simulink library "engine_AMT280_lib"  (Simulink 7.2)
settings: Solver=ode45  SolverMode=SingleTasking  StartTime=0.0  StopTime=10.0  RelTol=1e-3
libraries: simulink x1
settings Model: Creator=amurch  LastModifiedBy=amurch

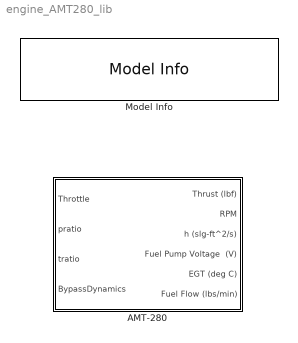
== system engine_AMT280_lib ==
  AMT-280 : Subsystem
      mask init:
      | % Curve fit parameters for AMT-280 Model
      | Coeff_thrust   = [ 5.7372e-05  -5.2629e-03   3.1586e-01  -5.1517e+00];
      | Coeff_throttle = [ -4.3078e-03   1.1110e+00   2.9012e+01];
      | Coeff_fuelflow = [ 1.0140e-04  -1.5867e-03   2.0125e-01];
      | Coeff_tau      = [ -2.2400e-02   2.9948e+00];
      | 
      | 
      | % Equvalent Shaft parameters for engine
      | shaft_dia = 0.75/12.0;       % diameter of rotating turbine in feet 
      | shaft_len = 6.25/12.0;       % length of rotating turbine in feet   
      | density   = 15.2;            % mass density of steel in slugs/ft^3 
      | 
      | fuelpump_table = [ 0.90 1.0 6.4]; %volts, table of fuel pump voltages  - not accurate at the moment 2-4-08
      | fuelflow_table = [0.00 0.1762 1.34044]; %lbs/min,   fuel flow rates corresponding to pump voltages (pumpv_table)
  Model Info : simulink/Model-Wide Utilities/Model Info  SystemSampleTime=-1  InitialBlockCM=None  BlockCM=None  Frame=on  DisplayStringWithTags=|  HorizontalTextAlignment=Center  LeftAlignmentValue=0.5  SourceBlockDiagram=engine_AMT280_lib  TagMaxNumber=20
      | AMT-280 Engine Library
      | 
      | Model Version: %<ModelVersion>
      | Last modifed by %<LastModifiedBy> on %<LastModificationDate>

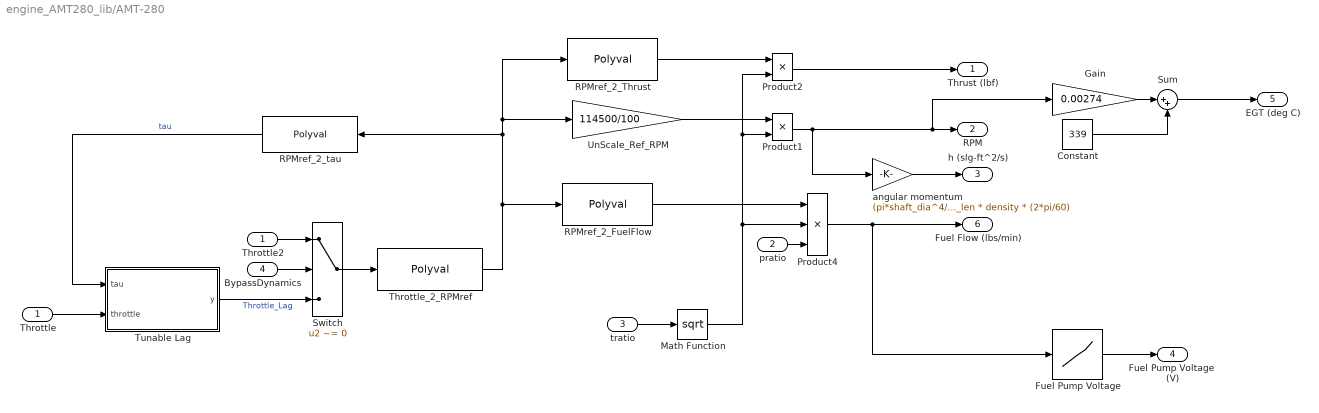
== system engine_AMT280_lib/AMT-280 ==
  Throttle : Inport  OutDataType=sfix(16)  OutScaling=2^0
  pratio : Inport  Port=2  OutDataType=sfix(16)  OutScaling=2^0
  tratio : Inport  Port=3  OutDataType=sfix(16)  OutScaling=2^0
  BypassDynamics : Inport  Port=4  OutDataType=sfix(16)  OutScaling=2^0
  Constant : Constant  Value=339  OutDataType=sfix(16)  OutScaling=2^0
  Fuel Pump Voltage : Lookup  InputValues=fuelflow_table  Table=fuelpump_table  LookUpMeth=Interpolation-Use End Values  OutDataType=sfix(16)  OutScaling=2^0
  Gain : Gain  Gain=0.00274  ParameterDataType=sfix(16)  ParameterScaling=2^0  OutDataType=sfix(16)  OutScaling=2^0
  Math Function : Math  Operator=sqrt  OutDataType=sfix(16)  OutScaling=2^0  SaturateOnIntegerOverflow=on
  Product1 : Product  OutDataType=sfix(16)  OutScaling=2^0  RndMeth=Zero
  Product2 : Product  OutDataType=sfix(16)  OutScaling=2^0  RndMeth=Zero
  Product4 : Product  Inputs=3  OutDataType=sfix(16)  OutScaling=2^0  RndMeth=Zero
  RPMref_2_FuelFlow : Polyval  Coefs=Coeff_fuelflow
  RPMref_2_Thrust : Polyval  Coefs=Coeff_thrust
  RPMref_2_tau : Polyval  Orientation=left  Coefs=Coeff_tau
  Sum : Sum  Inputs=|++  OutDataType=sfix(16)  OutScaling=2^0
  Switch : Switch  Criteria=u2 ~= 0
  Throttle2 : InportShadow  Port=1  OutDataType=sfix(16)  OutScaling=2^0  LatchByCopyingInsideSignal=off
  Throttle_2_RPMref : Polyval  Coefs=Coeff_throttle
  Tunable Lag : Subsystem
  UnScale_Ref_RPM : Gain  Gain=114500/100  ParameterDataType=sfix(16)  ParameterScaling=2^0  OutDataType=sfix(16)  OutScaling=2^0
  angular momentum : Gain  Gain=(pi*shaft_dia^4/32) * shaft_len * density * (2*pi/60)  ParameterDataType=sfix(16)  ParameterScaling=2^0  OutDataType=sfix(16)  OutScaling=2^0
  Thrust (lbf) : Outport  OutDataType=sfix(16)  OutScaling=2^0
  RPM : Outport  Port=2  OutDataType=sfix(16)  OutScaling=2^0
  h (slg-ft^2/s) : Outport  Port=3  OutDataType=sfix(16)  OutScaling=2^0
  Fuel Pump Voltage  (V) : Outport  Port=4  OutDataType=sfix(16)  OutScaling=2^0
  EGT (deg C) : Outport  Port=5  OutDataType=sfix(16)  OutScaling=2^0
  Fuel Flow (lbs/min) : Outport  Port=6  OutDataType=sfix(16)  OutScaling=2^0
  wires:
  RPMref_2_FuelFlow/1 -> Product4/1
  Product4/1 -> Fuel Flow (lbs/min)/1, Fuel Pump Voltage/1
  Product2/1 -> Thrust (lbf)/1
  Math Function/1 -> Product2/2, Product1/2, Product4/2
  RPMref_2_Thrust/1 -> Product2/1
  tratio/1 -> Math Function/1
  Product1/1 -> angular momentum/1, RPM/1, Gain/1
  pratio/1 -> Product4/3
  UnScale_Ref_RPM/1 -> Product1/1
  angular momentum/1 -> h (slg-ft^2/s)/1
  Throttle_2_RPMref/1 -> RPMref_2_tau/1, UnScale_Ref_RPM/1, RPMref_2_Thrust/1, RPMref_2_FuelFlow/1
  Throttle/1 -> Tunable Lag/2(throttle)
  RPMref_2_tau/1 -> Tunable Lag/1(tau)  "tau"
  Fuel Pump Voltage/1 -> Fuel Pump Voltage  (V)/1
  Sum/1 -> EGT (deg C)/1
  Constant/1 -> Sum/2
  Gain/1 -> Sum/1
  BypassDynamics/1 -> Switch/2
  Throttle2/1 -> Switch/1
  Tunable Lag/1(y) -> Switch/3  "Throttle_Lag"
  Switch/1 -> Throttle_2_RPMref/1

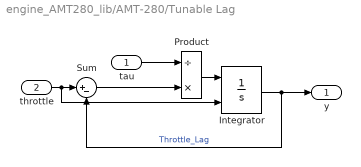
== system engine_AMT280_lib/AMT-280/Tunable Lag ==
  tau : Inport  OutDataType=sfix(16)  OutScaling=2^0
  throttle : Inport  Port=2  OutDataType=sfix(16)  OutScaling=2^0
  Integrator : Integrator  InitialConditionSource=external
  Product : Product  Inputs=/*  OutDataType=sfix(16)  OutScaling=2^0  RndMeth=Zero
  Sum : Sum  Inputs=|+-  OutDataType=sfix(16)  OutScaling=2^0
  y : Outport  OutDataType=sfix(16)  OutScaling=2^0
  wires:
  Integrator/1 -> Sum/2, y/1  "Throttle_Lag"
  Product/1 -> Integrator/1
  Sum/1 -> Product/2
  tau/1 -> Product/1
  throttle/1 -> Sum/1, Integrator/2
